simulink model "task2_2old"  (R2023a)
settings: Solver=VariableStepAuto  StartTime=0.0  StopTime=10.0  RelTol=1e-3
settings Model: Creator=user  LastModifiedBy=user

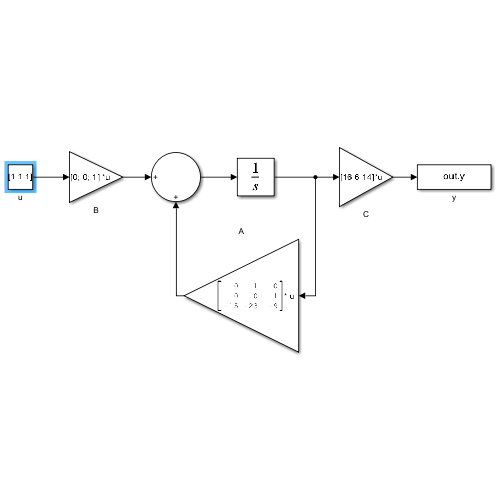
[thumbnail: Simulink's stored preview of the top-level diagram]
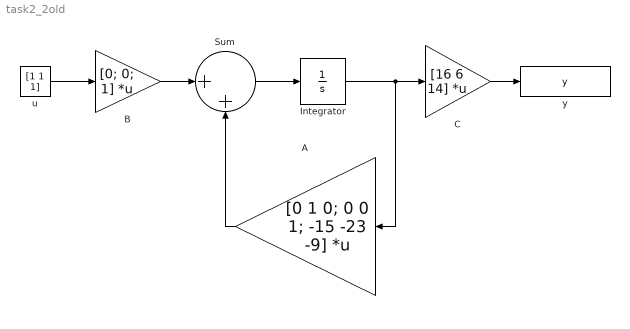
== system task2_2old ==
  A : Gain  Gain=[0 1 0; 0 0 1; -15 -23 -9]  Multiplication=Matrix(K*u)
  B : Gain  Gain=[0; 0; 1]  Multiplication=Matrix(K*u)
  C : Gain  Gain=[16 6 14]  Multiplication=Matrix(K*u)
  Integrator : Integrator
  Sum : Sum  Inputs=|++
  u : Constant  Value=[1 1 1]  VectorParams1D=off
  y : ToWorkspace  VariableName=y  SaveFormat=Timeseries  SampleTime=-1
  wires:
  u/1 -> B/1
  B/1 -> Sum/1
  Sum/1 -> Integrator/1
  Integrator/1 -> A/1, C/1
  C/1 -> y/1
  A/1 -> Sum/2
